simulink model "test"  (R2014b)
settings: Solver=ode45  StartTime=0.0  StopTime=10.0  RelTol=1e-3
settings Model: Creator=mshahria  LastModifiedBy=mshahria

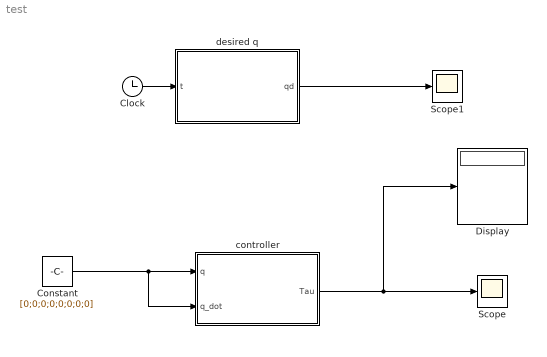
== system test ==
  Clock : Clock
  Constant : Constant  Value=[0;0;0;0;0;0;0;0]
  Display : Display
  Scope : Scope
  Scope1 : Scope
  controller : MATLAB Function  TreatAsAtomicUnit=on
  desired q : MATLAB Function  TreatAsAtomicUnit=on
  wires:
  Constant/1 -> controller/2(q_dot), controller/1(q)
  controller/1(Tau) -> Display/1, Scope/1
  Clock/1 -> desired q/1(t)
  desired q/1(qd) -> Scope1/1

== matlab function test/controller ==
  data: q input; Tau output; q_dot input
function Tau= fcn(q,q_dot)

theta_1= q(3);
theta_2= q(4);

theta_dot1=q(7);
theta_dot2=q(8);

x_dotdot=q_dot(5);
y_dotdot=q_dot(6);
theta_dotdot1=q_dot(7);
theta_dotdot2=q_dot(8);

% to avoid singularity on the docked mechanism:

if abs(theta_1-theta_2)<1e-2
    if theta_dot2>=0
     theta_2=theta_1+0.01;
    else
     theta_2=theta_1-0.01;
    end
end

%---------------------------------------------

Tau=Tau_computed(theta_1,theta_2,theta_dot1,theta_dot2,theta_dotdot1,theta_dotdot2,x_dotdot,y_dotdot);

== matlab function test/desired q ==
  data: t input; qd output
function qd= fcn(t)

qd=q_desired(t)
